simulink model "Lab_5"  (R2017b)
settings: Solver=VariableStepAuto  StartTime=0.0  StopTime=inf  MaxStep=0.1
values from neighbouring files (symbols this model uses):
  a = (r_a + r_p)/2    (= 7975.5)    [main.m]
  A_i = [A_i_1, A_i_2, A_i_3]    [main.m]
  alpha_m = deg2rad(11)    [main.m]
  C_d = 2.2    [main.m]
  DCM_0 = eye(3)    [main.m]
  dim = [w, l, h]    [main.m]
  i = 0    [main.m]
  I_1 = M/12 * (w^2 + l^2)    (= 0.0153029225)    [main.m]
  I_2 = M/12 * (w^2 + h^2)    (= 0.0314850625)    [main.m]
  I_3 = M/12 * (l^2 + h^2)    (= 0.041787985)    [main.m]
  m_m = (a_m^3*H_0)*(4*pi/mu_0)    [main.m]
  mu = 398600    [main.m]
  n = 2*pi/(60*60*24*365)    (= 1.99238499086e-07)    [main.m]
  OMG = 0    [main.m]
  omg = 0    [main.m]
  phi_0 = 0.1    [main.m]
  psi_0 = 0.1    [main.m]
  q_0 = [0 1/sqrt(3) 1/sqrt(3) 1/sqrt(3)]    [main.m]
  q_c = [0 0 0 1]'    [main.m]
  R_e = 6.378e+03    (= 6378)    [main.m]
  rho_d = 0.1    [main.m]
  rho_s = 0.5    [main.m]
  theta = 0    [main.m]
  theta_0 = 0.1    [main.m]
  w1_0 = 0    [main.m]
  w2_0 = 0    [main.m]
  w3_0 = (sqrt(mu/(7.9755e+03)^3))/10    [main.m]
  w_e = [0 0 0.00007291]    [main.m]
libraries: simulink x2, vrlib x2, dspmathops x2, sharedutil x1
settings Model: Creator=fcuzzocrea  LastModifiedBy=fcuzzocrea

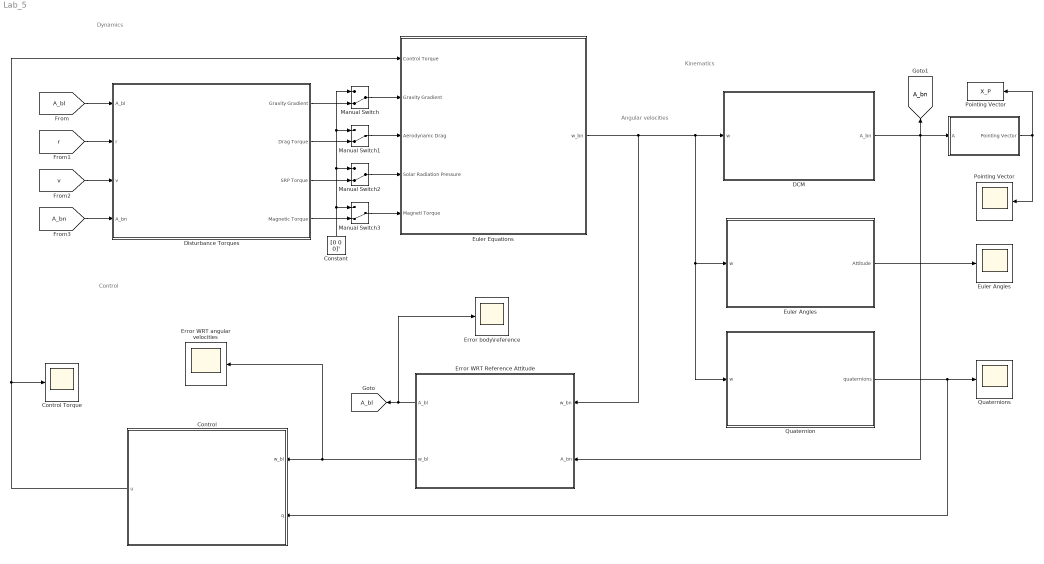
== system Lab_5 ==
  note: Control
  note: Dynamics
  note: Kinematics
  note: Angular velocities
  " " : Subsystem
  Constant : Constant  Value=[0 0 0]'
  Control : Subsystem
  "Control Torque " : Scope
  DCM : Subsystem
  Disturbance Torques : Subsystem
  "Error WRT Reference Attitude " : Subsystem
  Error WRT angular velocities : Scope
  "Error body\\reference  " : Scope
  "Euler Angles " : Subsystem
  "Euler Angles " : Scope
  "Euler Equations " : Subsystem
  Manual Switch{,1..3} (4 alike) : ManualSwitch  CurrentSetting=0
  Pointing Vector : Scope
  "Pointing Vector " : ToWorkspace  VariableName=X_P  SampleTime=-1
  Quaternion : Subsystem
  "Quaternions " : Scope
  tag scope: A_bl=global, A_bn=global
  wires:
  DCM/1(A_bn) -> [A_bn], "Error WRT Reference Attitude "/2(A_bn), " "/1(A)
  " "/1("Pointing Vector ") -> Pointing Vector/1, "Pointing Vector "/1
  "Euler Angles "/1(Attitude) -> "Euler Angles "/1
  "Euler Equations "/1(w_bn) -> "Error WRT Reference Attitude "/1(w_bn), Quaternion/1(w), "Euler Angles "/1(w), DCM/1(w)
  [A_bl] -> Disturbance Torques/1(A_bl)
  [r] -> Disturbance Torques/2(r)
  Manual Switch/1 -> "Euler Equations "/2(Gravity Gradient)
  Disturbance Torques/1("Gravity Gradient ") -> Manual Switch/2
  Constant/1 -> Manual Switch3/1, Manual Switch/1, Manual Switch1/1, Manual Switch2/1
  Quaternion/1(quaternions) -> Control/2(q), "Quaternions "/1
  [v] -> Disturbance Torques/3(v)
  [A_bn] -> Disturbance Torques/4(A_bn)
  Disturbance Torques/2(Drag Torque) -> Manual Switch1/2
  Manual Switch1/1 -> "Euler Equations "/3(Aerodynamc Drag)
  Disturbance Torques/3(SRP Torque) -> Manual Switch2/2
  Manual Switch2/1 -> "Euler Equations "/4(Solar Radiation Pressure)
  Manual Switch3/1 -> "Euler Equations "/5(Magneti Torque)
  Disturbance Torques/4(Magnetic Torque) -> Manual Switch3/2
  "Error WRT Reference Attitude "/1(A_bl) -> "Error body\\reference  "/1, [A_bl]
  "Error WRT Reference Attitude "/2(w_bl) -> Error WRT angular velocities/1, Control/1(w_bl)
  Control/1(u) -> "Control Torque "/1, "Euler Equations "/1(Control Torque)

== system Lab_5/  ==
  A : Inport
  Constant3 : Constant  Value=[1 0 0]'  VectorParams1D=off
  Math Function : Math  Operator=transpose  SaturateOnIntegerOverflow=on
  Product1 : Product  Multiplication=Matrix(*)
  "Pointing Vector " : Outport
  wires:
  Constant3/1 -> Product1/2
  Math Function/1 -> Product1/1
  A/1 -> Math Function/1
  Product1/1 -> "Pointing Vector "/1

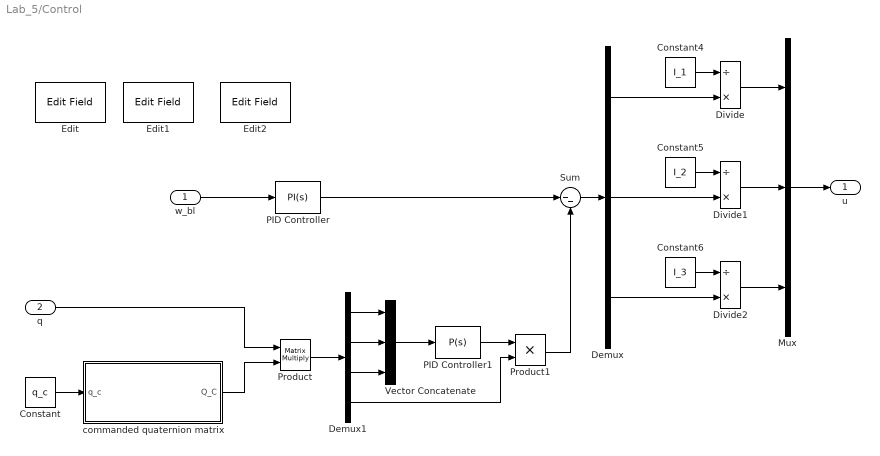
== system Lab_5/Control ==
  w_bl : Inport
  q : Inport  Port=2
  Constant : Constant  Value=q_c
  Constant4 : Constant  Value=I_1
  Constant5 : Constant  Value=I_2
  Constant6 : Constant  Value=I_3
  Demux : Demux  Outputs=3
  Demux1 : Demux
  Divide : Product  Inputs=/*
  Divide1 : Product  Inputs=/*
  Divide2 : Product  Inputs=/*
  Edit : EditField  WebBlockId=947  ModelName=Lab_5  LabelPosition=Hide  ShowInitialText=off  Alignment=Center
  Edit1 : EditField  WebBlockId=948  ModelName=Lab_5  LabelPosition=Hide  ShowInitialText=off  Alignment=Center
  Edit2 : EditField  WebBlockId=949  ModelName=Lab_5  LabelPosition=Hide  ShowInitialText=off  Alignment=Center
  Mux : Mux  Inputs=3
  PID Controller : simulink/Continuous/PID Controller  Controller=PI  TimeDomain=Continuous-time  SampleTime=-1  IntegratorMethod=Forward Euler  FilterMethod=Forward Euler  Form=Parallel  UseFilter=on  ControllerParametersSource=internal  P=1.1  I=0.3  D=0  N=100  InitialConditionSource=internal  InitialConditionForIntegrator=0  InitialConditionForFilter=0  ExternalReset=none  LimitOutput=off  UpperSaturationLimit=inf  LowerSaturationLimit=-inf  LinearizeAsGain=on  AntiWindupMode=none  Kb=1  TrackingMode=off  Kt=1  PParamMin=[]  PParamMax=[]  IParamMin=[]  IParamMax=[]  DParamMin=[]  DParamMax=[]  NParamMin=[]  NParamMax=[]  KbParamMin=[]  KbParamMax=[]  KtParamMin=[]  KtParamMax=[]  POutMin=[]  POutMax=[]  IOutMin=[]  IOutMax=[]  DOutMin=[]  DOutMax=[]  NOutMin=[]  NOutMax=[]  KbOutMin=[]  KbOutMax=[]  KtOutMin=[]  KtOutMax=[]  IntegratorOutMin=[]  IntegratorOutMax=[]  FilterOutMin=[]  FilterOutMax=[]  SumOutMin=[]  SumOutMax=[]  SumI1OutMin=[]  SumI1OutMax=[]  SumI2OutMin=[]  SumI2OutMax=[]  SumI3OutMin=[]  SumI3OutMax=[]  SumDOutMin=[]  SumDOutMax=[]  SaturationOutMin=[]  SaturationOutMax=[]  IntegratorContinuousStateAttributes=''  IntegratorStateMustResolveToSignalObject=off  IntegratorRTWStateStorageClass=Auto  FilterContinuousStateAttributes=''  FilterStateMustResolveToSignalObject=off  FilterRTWStateStorageClass=Auto  DifferentiatorICPrevScaledInput=0  DifferentiatorOutMin=[]  DifferentiatorOutMax=[]  InitialConditionSetting=State (most efficient)  FilterDiffOutCoefMin=[]  FilterDiffOutCoefMax=[]  SumDenOutMin=[]  SumDenOutMax=[]  SumNumOutMin=[]  SumNumOutMax=[]  ReciprocalOutMin=[]  ReciprocalOutMax=[]  DivideOutMin=[]  DivideOutMax=[]  TunerSelectOption=Transfer Function Based (PID Tuner App)
  PID Controller1 : simulink/Continuous/PID Controller  Controller=P  TimeDomain=Continuous-time  SampleTime=-1  IntegratorMethod=Forward Euler  FilterMethod=Forward Euler  Form=Parallel  UseFilter=on  ControllerParametersSource=internal  P=0.001  I=0.1e-3  D=0  N=100  InitialConditionSource=internal  InitialConditionForIntegrator=0  InitialConditionForFilter=0  ExternalReset=none  LimitOutput=off  UpperSaturationLimit=inf  LowerSaturationLimit=-inf  LinearizeAsGain=on  AntiWindupMode=none  Kb=1  TrackingMode=off  Kt=1  PParamMin=[]  PParamMax=[]  IParamMin=[]  IParamMax=[]  DParamMin=[]  DParamMax=[]  NParamMin=[]  NParamMax=[]  KbParamMin=[]  KbParamMax=[]  KtParamMin=[]  KtParamMax=[]  POutMin=[]  POutMax=[]  IOutMin=[]  IOutMax=[]  DOutMin=[]  DOutMax=[]  NOutMin=[]  NOutMax=[]  KbOutMin=[]  KbOutMax=[]  KtOutMin=[]  KtOutMax=[]  IntegratorOutMin=[]  IntegratorOutMax=[]  FilterOutMin=[]  FilterOutMax=[]  SumOutMin=[]  SumOutMax=[]  SumI1OutMin=[]  SumI1OutMax=[]  SumI2OutMin=[]  SumI2OutMax=[]  SumI3OutMin=[]  SumI3OutMax=[]  SumDOutMin=[]  SumDOutMax=[]  SaturationOutMin=[]  SaturationOutMax=[]  IntegratorContinuousStateAttributes=''  IntegratorStateMustResolveToSignalObject=off  IntegratorRTWStateStorageClass=Auto  FilterContinuousStateAttributes=''  FilterStateMustResolveToSignalObject=off  FilterRTWStateStorageClass=Auto  DifferentiatorICPrevScaledInput=0  DifferentiatorOutMin=[]  DifferentiatorOutMax=[]  InitialConditionSetting=State (most efficient)  FilterDiffOutCoefMin=[]  FilterDiffOutCoefMax=[]  SumDenOutMin=[]  SumDenOutMax=[]  SumNumOutMin=[]  SumNumOutMax=[]  ReciprocalOutMin=[]  ReciprocalOutMax=[]  DivideOutMin=[]  DivideOutMax=[]  TunerSelectOption=Transfer Function Based (PID Tuner App)
  Product : Product  Multiplication=Matrix(*)
  Product1 : Product
  Sum : Sum  Inputs=|--
  Vector Concatenate : Concatenate  NumInputs=3
  commanded quaternion matrix : MATLAB Function  TreatAsAtomicUnit=on
  u : Outport
  wires:
  w_bl/1 -> PID Controller/1
  Divide/1 -> Mux/1
  Constant4/1 -> Divide/1
  Constant5/1 -> Divide1/1
  Divide1/1 -> Mux/2
  Constant6/1 -> Divide2/1
  Divide2/1 -> Mux/3
  Demux/2 -> Divide1/2
  Demux/1 -> Divide/2
  Mux/1 -> u/1
  Demux/3 -> Divide2/2
  Constant/1 -> commanded quaternion matrix/1(q_c)
  q/1 -> Product/1
  commanded quaternion matrix/1(Q_C) -> Product/2
  PID Controller/1 -> Sum/1
  Sum/1 -> Demux/1
  Product/1 -> Demux1/1
  Demux1/4 -> Product1/2
  Demux1/1 -> Vector Concatenate/1
  Demux1/2 -> Vector Concatenate/2
  Demux1/3 -> Vector Concatenate/3
  Vector Concatenate/1 -> PID Controller1/1
  PID Controller1/1 -> Product1/1
  Product1/1 -> Sum/2

== system Lab_5/DCM ==
  w : Inport  Unit=rad/s  PortDimensions=3
  fromBodyToEarth : Subsystem
  A_bn : Outport
  wires:
  w/1 -> fromBodyToEarth/1("w ")
  fromBodyToEarth/1(A_bn) -> A_bn/1

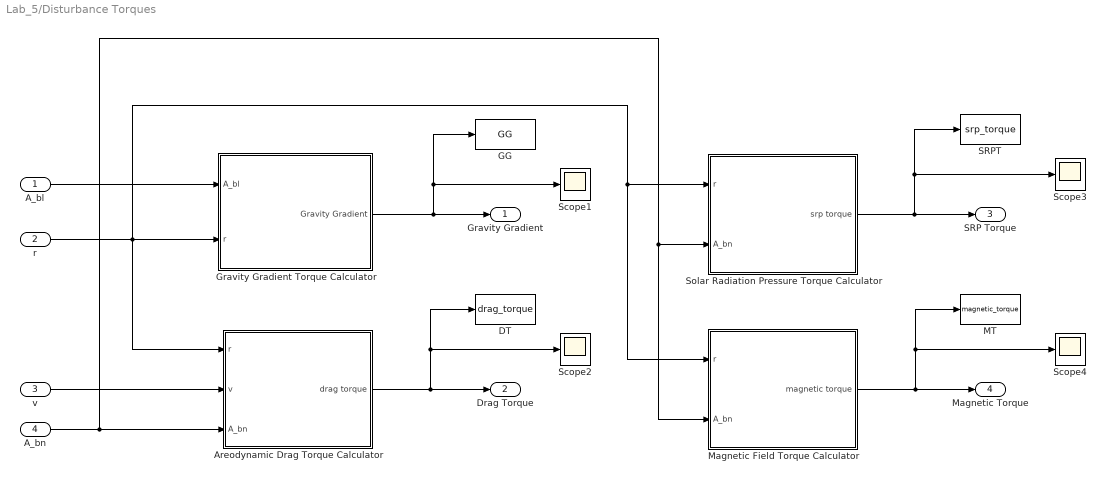
== system Lab_5/Disturbance Torques ==
  A_bl : Inport
  r : Inport  Port=2
  v : Inport  Port=3
  A_bn : Inport  Port=4
  "Areodynamic Drag Torque Calculator " : Subsystem
  DT : ToWorkspace  VariableName=drag_torque  SampleTime=-1
  GG : ToWorkspace  VariableName=GG  SampleTime=-1
  Gravity Gradient Torque Calculator : Subsystem
  MT : ToWorkspace  VariableName=magnetic_torque  SampleTime=-1
  Magnetic Field Torque Calculator : Subsystem
  SRPT : ToWorkspace  VariableName=srp_torque  SampleTime=-1
  Scope{1..4} (4 alike) : Scope
  Solar Radiation Pressure Torque Calculator : Subsystem
  "Gravity Gradient " : Outport
  Drag Torque : Outport  Port=2
  SRP Torque : Outport  Port=3
  Magnetic Torque : Outport  Port=4
  wires:
  A_bl/1 -> Gravity Gradient Torque Calculator/1(A_bl)
  Gravity Gradient Torque Calculator/1(Gravity Gradient) -> GG/1, Scope1/1, "Gravity Gradient "/1
  v/1 -> "Areodynamic Drag Torque Calculator "/2(v)
  A_bn/1 -> Magnetic Field Torque Calculator/2(A_bn), Solar Radiation Pressure Torque Calculator/2(A_bn), "Areodynamic Drag Torque Calculator "/3(A_bn)
  "Areodynamic Drag Torque Calculator "/1("drag torque ") -> DT/1, Scope2/1, Drag Torque/1
  Solar Radiation Pressure Torque Calculator/1("srp torque ") -> SRP Torque/1, Scope3/1, SRPT/1
  Magnetic Field Torque Calculator/1("magnetic torque ") -> Magnetic Torque/1, Scope4/1, MT/1
  r/1 -> "Areodynamic Drag Torque Calculator "/1(r), Gravity Gradient Torque Calculator/2(r), Magnetic Field Torque Calculator/1(r), Solar Radiation Pressure Torque Calculator/1(r)

== system Lab_5/Error WRT Reference Attitude  ==
  note: Error on angular velocities
  note: Error on reference frames
  note: OSS : Reference frame here stands for frame that we wan to track, don't make confusion
  w_bn : Inport
  A_bn : Inport  Port=2
  Angular velocity of the orbital pointing frame : Subsystem
  Relative angular velocities between the body frame and the orbital pointing frame (the error in terms of angular velocities). : Subsystem
  Rotation matrix between the body frame and the orbital pointing frame (the error on pointing) : Subsystem
  To Workspace : ToWorkspace  VariableName=w_bl  SampleTime=-1
  A_bl : Outport
  w_bl : Outport  Port=2
  wires:
  A_bn/1 -> Rotation matrix between the body frame and the orbital pointing frame (the error on pointing)/1("A_bn ")
  w_bn/1 -> Relative angular velocities between the body frame and the orbital pointing frame (the error in terms of angular velocities)./1(w_bn)
  Rotation matrix between the body frame and the orbital pointing frame (the error on pointing)/1("A_bl ") -> A_bl/1, Relative angular velocities between the body frame and the orbital pointing frame (the error in terms of angular velocities)./2("A_bl ")
  Angular velocity of the orbital pointing frame/1(w_ln) -> Relative angular velocities between the body frame and the orbital pointing frame (the error in terms of angular velocities)./3("w_ln ")
  Relative angular velocities between the body frame and the orbital pointing frame (the error in terms of angular velocities)./1(w_bl) -> To Workspace/1, w_bl/1

== system Lab_5/Euler Angles  ==
  w : Inport
  Demux : Demux  Outputs=3
  Integrator : Integrator  InitialCondition=phi_0
  Integrator1 : Integrator  InitialCondition=theta_0
  Integrator2 : Integrator  InitialCondition=psi_0
  MATLAB Function : MATLAB Function  TreatAsAtomicUnit=on
  Mux : Mux  Inputs=3
  Attitude : Outport
  wires:
  Demux/1 -> MATLAB Function/1(w1)
  Demux/2 -> MATLAB Function/2(w2)
  Demux/3 -> MATLAB Function/3(w3)
  MATLAB Function/1(phi_dot) -> Integrator/1
  MATLAB Function/2(tetha_dot) -> Integrator1/1
  MATLAB Function/3(psi_dot) -> Integrator2/1
  Integrator/1 -> Mux/1
  Integrator1/1 -> Mux/2, MATLAB Function/4(tetha)
  Mux/1 -> Attitude/1
  Integrator2/1 -> MATLAB Function/5(psi), Mux/3
  w/1 -> Demux/1

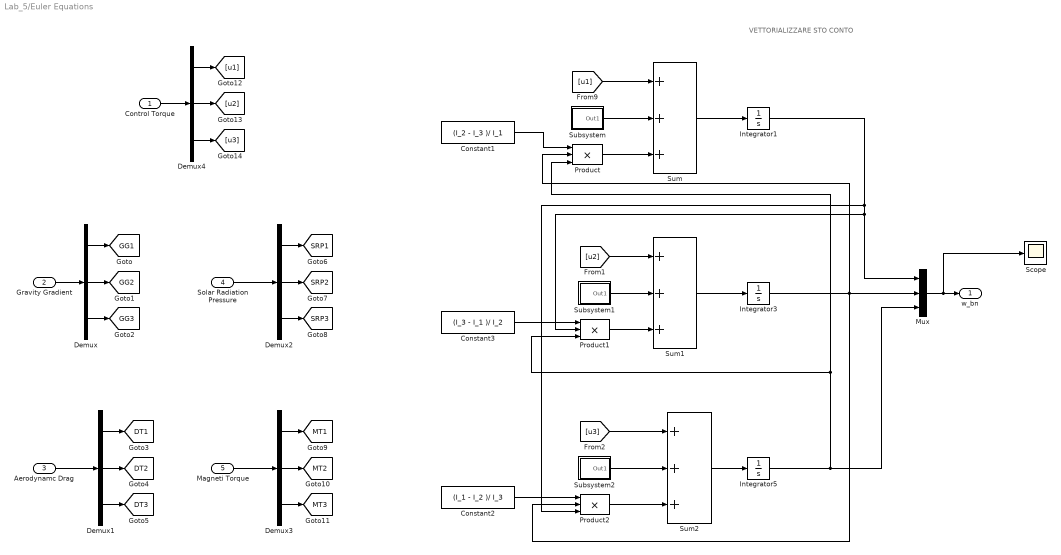
== system Lab_5/Euler Equations  ==
  note: VETTORIALIZZARE STO CONTO
  Control Torque : Inport
  Gravity Gradient : Inport  Port=2
  Aerodynamc Drag : Inport  Port=3
  Solar Radiation Pressure : Inport  Port=4
  Magneti Torque : Inport  Port=5
  Constant1 : Constant  Value=(I_2 - I_3 )/ I_1
  Constant2 : Constant  Value=(I_1 - I_2 )/ I_3
  Constant3 : Constant  Value=(I_3 - I_1 )/ I_2
  Demux{,1..4} (5 alike) : Demux  Outputs=3
  Integrator1 : Integrator  InitialCondition=w1_0
  Integrator3 : Integrator  InitialCondition=w2_0
  Integrator5 : Integrator  InitialCondition=w3_0
  Mux : Mux  Inputs=3
  Product : Product  Inputs=3
  Product1 : Product  Inputs=3
  Product2 : Product  Inputs=3
  Scope : Scope
  Subsystem : Subsystem
  Subsystem1 : Subsystem
  Subsystem2 : Subsystem
  Sum : Sum  Inputs=+++
  Sum1 : Sum  Inputs=+++
  Sum2 : Sum  Inputs=+++
  w_bn : Outport  Unit=rad/s  PortDimensions=3
  tag scope: DT1=global, DT2=global, DT3=global, GG1=global, GG2=global, GG3=global, MT1=global, MT2=global, MT3=global, SRP1=global, SRP2=global, SRP3=global
  wires:
  Integrator3/1 -> Product2/2, Mux/2, Product/2
  Integrator5/1 -> Product/3, Product1/3, Mux/3
  Constant1/1 -> Product/1
  Constant3/1 -> Product1/1
  Constant2/1 -> Product2/1
  Integrator1/1 -> Mux/1, Product1/2, Product2/3
  Mux/1 -> w_bn/1, Scope/1
  Gravity Gradient/1 -> Demux/1
  Demux/1 -> [GG1]
  Demux/2 -> [GG2]
  Demux/3 -> [GG3]
  Demux1/3 -> [DT3]
  Aerodynamc Drag/1 -> Demux1/1
  Demux1/2 -> [DT2]
  Demux1/1 -> [DT1]
  Demux2/3 -> [SRP3]
  Solar Radiation Pressure/1 -> Demux2/1
  Demux2/1 -> [SRP1]
  Demux2/2 -> [SRP2]
  Demux3/2 -> [MT2]
  Demux3/3 -> [MT3]
  Demux3/1 -> [MT1]
  Magneti Torque/1 -> Demux3/1
  Demux4/1 -> [u1]
  Demux4/3 -> [u3]
  Control Torque/1 -> Demux4/1
  Demux4/2 -> [u2]
  Subsystem/1(Out1) -> Sum/2
  Product/1 -> Sum/3
  Sum/1 -> Integrator1/1
  Sum1/1 -> Integrator3/1
  Product1/1 -> Sum1/3
  Subsystem1/1(Out1) -> Sum1/2
  Sum2/1 -> Integrator5/1
  Product2/1 -> Sum2/3
  Subsystem2/1(Out1) -> Sum2/2
  [u1] -> Sum/1
  [u3] -> Sum2/1
  [u2] -> Sum1/1

== system Lab_5/Quaternion ==
  w : Inport
  Integrator2 : Integrator  InitialCondition=q_0
  Quaternion kinematics : MATLAB Function  TreatAsAtomicUnit=on
  quaternions : Outport
  wires:
  Integrator2/1 -> quaternions/1, Quaternion kinematics/1(q)  "q"
  Quaternion kinematics/1(dq) -> Integrator2/1  "dq"
  w/1 -> Quaternion kinematics/2(omega)  "ω_b"

== system Lab_5/DCM/fromBodyToEarth ==
  "w " : Inport
  "Assembly [w^] " : Subsystem
  Demux : Demux  Outputs=3
  Integrator : Integrator  InitialCondition=DCM_0
  MATLAB Function1 : MATLAB Function  TreatAsAtomicUnit=on
  Product : Product  Multiplication=Matrix(*)
  A_bn : Outport
  wires:
  Product/1 -> Integrator/1
  Integrator/1 -> A_bn/1, MATLAB Function1/1(u)
  "w "/1 -> Demux/1
  Demux/1 -> "Assembly [w^] "/1(w1)
  Demux/2 -> "Assembly [w^] "/2(w2)
  Demux/3 -> "Assembly [w^] "/3(w3)
  "Assembly [w^] "/1(-[w]^) -> Product/1
  MATLAB Function1/1(y) -> Product/2

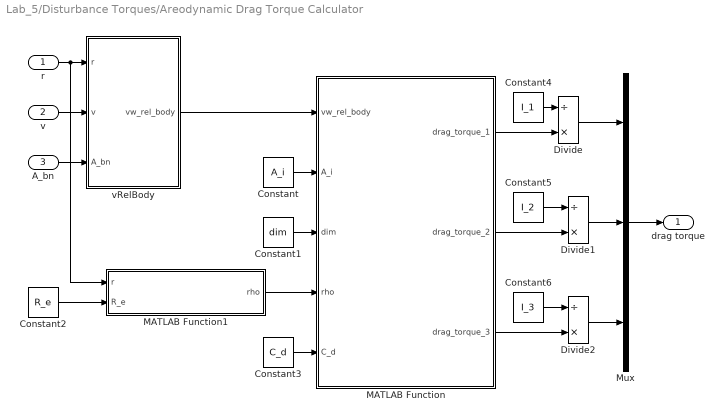
== system Lab_5/Disturbance Torques/Areodynamic Drag Torque Calculator  ==
  r : Inport
  v : Inport  Port=2
  A_bn : Inport  Port=3
  Constant : Constant  Value=A_i
  Constant1 : Constant  Value=dim
  Constant2 : Constant  Value=R_e
  Constant3 : Constant  Value=C_d
  Constant4 : Constant  Value=I_1
  Constant5 : Constant  Value=I_2
  Constant6 : Constant  Value=I_3
  Divide : Product  Inputs=/*
  Divide1 : Product  Inputs=/*
  Divide2 : Product  Inputs=/*
  MATLAB Function : MATLAB Function  TreatAsAtomicUnit=on
  MATLAB Function1 : MATLAB Function  TreatAsAtomicUnit=on
  Mux : Mux  Inputs=3
  vRelBody : Subsystem
  "drag torque " : Outport
  wires:
  r/1 -> MATLAB Function1/1(r), vRelBody/1(r)
  v/1 -> vRelBody/2(v)
  A_bn/1 -> vRelBody/3(A_bn)
  vRelBody/1(vw_rel_body) -> MATLAB Function/1(vw_rel_body)
  Constant/1 -> MATLAB Function/2(A_i)
  Constant1/1 -> MATLAB Function/3(dim)
  Constant3/1 -> MATLAB Function/5(C_d)
  Mux/1 -> "drag torque "/1
  MATLAB Function/1(drag_torque_1) -> Divide/2
  Divide/1 -> Mux/1
  Constant4/1 -> Divide/1
  Constant5/1 -> Divide1/1
  MATLAB Function/2(drag_torque_2) -> Divide1/2
  Divide1/1 -> Mux/2
  Constant6/1 -> Divide2/1
  MATLAB Function/3(drag_torque_3) -> Divide2/2
  Divide2/1 -> Mux/3
  Constant2/1 -> MATLAB Function1/2(R_e)
  MATLAB Function1/1(rho) -> MATLAB Function/4(rho)

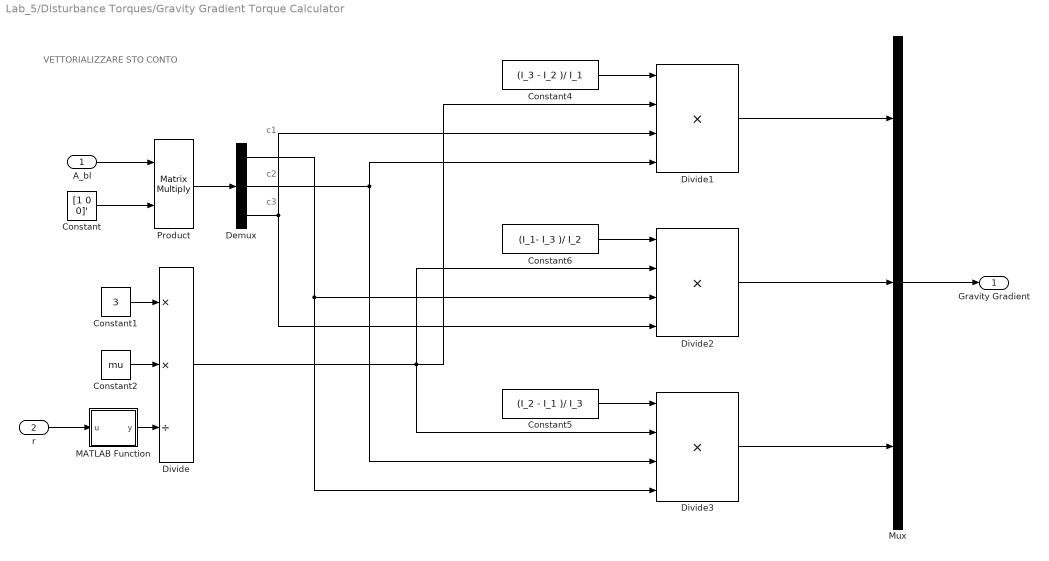
== system Lab_5/Disturbance Torques/Gravity Gradient Torque Calculator ==
  note: VETTORIALIZZARE STO CONTO
  note: c2
  note: c3
  note: c1
  A_bl : Inport
  r : Inport  Port=2
  Constant : Constant  Value=[1 0 0]'
  Constant1 : Constant  Value=3
  Constant2 : Constant  Value=mu
  Constant4 : Constant  Value=(I_3 - I_2 )/ I_1
  Constant5 : Constant  Value=(I_2 - I_1 )/ I_3
  Constant6 : Constant  Value=(I_1- I_3 )/ I_2
  Demux : Demux  Outputs=3
  Divide : Product  Inputs=**/
  Divide1 : Product  Inputs=****
  Divide2 : Product  Inputs=****
  Divide3 : Product  Inputs=****
  MATLAB Function : MATLAB Function  TreatAsAtomicUnit=on
  Mux : Mux  Inputs=3
  Product : Product  Multiplication=Matrix(*)
  Gravity Gradient : Outport
  wires:
  Demux/3 -> Divide2/4, Divide1/3
  Constant1/1 -> Divide/1
  r/1 -> MATLAB Function/1(u)
  Constant5/1 -> Divide3/1
  Divide/1 -> Divide3/2, Divide1/2, Divide2/2
  Demux/1 -> Divide3/4, Divide2/3
  Demux/2 -> Divide3/3, Divide1/4
  Product/1 -> Demux/1
  Constant6/1 -> Divide2/1
  A_bl/1 -> Product/1
  Constant4/1 -> Divide1/1
  MATLAB Function/1(y) -> Divide/3
  Constant/1 -> Product/2
  Constant2/1 -> Divide/2
  Divide1/1 -> Mux/1
  Divide2/1 -> Mux/2
  Divide3/1 -> Mux/3
  Mux/1 -> Gravity Gradient/1

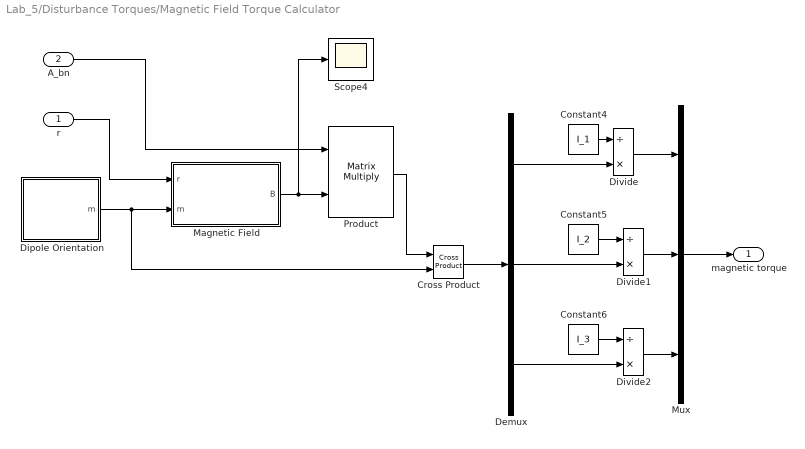
== system Lab_5/Disturbance Torques/Magnetic Field Torque Calculator ==
  r : Inport
  A_bn : Inport  Port=2
  Constant4 : Constant  Value=I_1
  Constant5 : Constant  Value=I_2
  Constant6 : Constant  Value=I_3
  Cross Product : vrlib/Utilities/Cross Product
      settings: SourceProductBaseCode=VR
  Demux : Demux  Outputs=3
  Dipole Orientation : Subsystem
  Divide : Product  Inputs=/*
  Divide1 : Product  Inputs=/*
  Divide2 : Product  Inputs=/*
  Magnetic Field : Subsystem
  Mux : Mux  Inputs=3
  Product : Product  Multiplication=Matrix(*)
  Scope4 : Scope
  "magnetic torque " : Outport
  wires:
  r/1 -> Magnetic Field/1(r)
  Demux/3 -> Divide2/2
  Mux/1 -> "magnetic torque "/1
  A_bn/1 -> Product/1
  Constant4/1 -> Divide/1
  Demux/2 -> Divide1/2
  Constant5/1 -> Divide1/1
  Demux/1 -> Divide/2
  Divide/1 -> Mux/1
  Product/1 -> Cross Product/1
  Divide1/1 -> Mux/2
  Cross Product/1 -> Demux/1
  Divide2/1 -> Mux/3
  Constant6/1 -> Divide2/1
  Magnetic Field/1("B ") -> Scope4/1, Product/2
  Dipole Orientation/1(m) -> Cross Product/2, Magnetic Field/2(m)

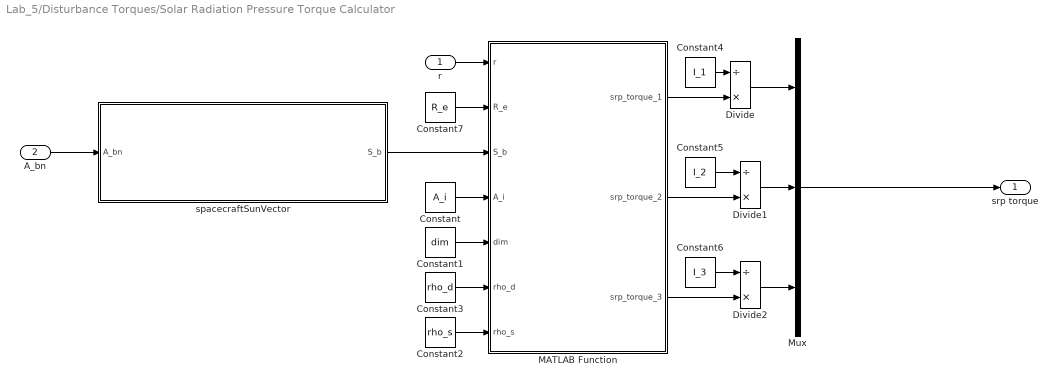
== system Lab_5/Disturbance Torques/Solar Radiation Pressure Torque Calculator ==
  r : Inport
  A_bn : Inport  Port=2
  Constant : Constant  Value=A_i
  Constant1 : Constant  Value=dim
  Constant2 : Constant  Value=rho_s
  Constant3 : Constant  Value=rho_d
  Constant4 : Constant  Value=I_1
  Constant5 : Constant  Value=I_2
  Constant6 : Constant  Value=I_3
  Constant7 : Constant  Value=R_e
  Divide : Product  Inputs=/*
  Divide1 : Product  Inputs=/*
  Divide2 : Product  Inputs=/*
  MATLAB Function : MATLAB Function  TreatAsAtomicUnit=on
  Mux : Mux  Inputs=3
  spacecraftSunVector : Subsystem
  "srp torque " : Outport
  wires:
  A_bn/1 -> spacecraftSunVector/1(A_bn)
  spacecraftSunVector/1("S_b ") -> MATLAB Function/3(S_b)
  Constant/1 -> MATLAB Function/4(A_i)
  Constant1/1 -> MATLAB Function/5(dim)
  Constant3/1 -> MATLAB Function/6(rho_d)
  Constant2/1 -> MATLAB Function/7(rho_s)
  MATLAB Function/3(srp_torque_3) -> Divide2/2
  Divide/1 -> Mux/1
  MATLAB Function/2(srp_torque_2) -> Divide1/2
  Constant5/1 -> Divide1/1
  Constant6/1 -> Divide2/1
  MATLAB Function/1(srp_torque_1) -> Divide/2
  Divide1/1 -> Mux/2
  Constant4/1 -> Divide/1
  Mux/1 -> "srp torque "/1
  Divide2/1 -> Mux/3
  r/1 -> MATLAB Function/1(r)
  Constant7/1 -> MATLAB Function/2(R_e)

== system Lab_5/Error WRT Reference Attitude /Angular velocity of the orbital pointing frame ==
  Derivative : Derivative
  MATLAB Function : MATLAB Function  TreatAsAtomicUnit=on
  Math Function : Math  Operator=transpose  SaturateOnIntegerOverflow=on
  Product : Product  Multiplication=Matrix(*)
  w_ln : Outport
  wires:
  [A_ln] -> Math Function/1, Derivative/1
  Math Function/1 -> Product/2
  Derivative/1 -> Product/1
  Product/1 -> MATLAB Function/1(w_ln_cross)
  MATLAB Function/1(w_ln) -> w_ln/1

== system Lab_5/Error WRT Reference Attitude /Relative angular velocities between the body frame and the orbital pointing frame (the error in terms of angular velocities). ==
  w_bn : Inport
  "A_bl " : Inport  Port=2
  "w_ln " : Inport  Port=3
  Product : Product  Multiplication=Matrix(*)
  Subtract : Sum  Inputs=+-
  w_bl : Outport
  wires:
  Product/1 -> Subtract/2
  Subtract/1 -> w_bl/1
  w_bn/1 -> Subtract/1
  "A_bl "/1 -> Product/1
  "w_ln "/1 -> Product/2

== system Lab_5/Error WRT Reference Attitude /Rotation matrix between the body frame and the orbital pointing frame (the error on pointing) ==
  note: NB : La DCM è A_bn, per cui moltiplicando A_ln * A_bn becco A_bl !!!!
  note: Reference Attitude
  "A_bn " : Inport
  Math Function1 : Math  Operator=transpose  SaturateOnIntegerOverflow=on
  Product : Product  Multiplication=Matrix(*)
  Rotation matrix between the pointing orbital frame and the inertial frame : Subsystem
  "A_bl " : Outport
  wires:
  "A_bn "/1 -> Product/1
  Rotation matrix between the pointing orbital frame and the inertial frame/1("A_L\\N ") -> Math Function1/1
  Product/1 -> "A_bl "/1
  Math Function1/1 -> Product/2

== system Lab_5/Euler Equations /Subsystem ==
  Sum : Sum  Inputs=++++
  Out1 : Outport
  wires:
  Sum/1 -> Out1/1
  [GG1] -> Sum/4
  [DT1] -> Sum/3
  [SRP1] -> Sum/2
  [MT1] -> Sum/1

== system Lab_5/Euler Equations /Subsystem1 ==
  Sum2 : Sum  Inputs=++++
  Out1 : Outport
  wires:
  Sum2/1 -> Out1/1
  [GG2] -> Sum2/4
  [DT2] -> Sum2/3
  [SRP2] -> Sum2/2
  [MT2] -> Sum2/1

== system Lab_5/Euler Equations /Subsystem2 ==
  Sum3 : Sum  Inputs=++++
  Out1 : Outport
  wires:
  Sum3/1 -> Out1/1
  [GG3] -> Sum3/4
  [DT3] -> Sum3/3
  [SRP3] -> Sum3/2
  [MT3] -> Sum3/1

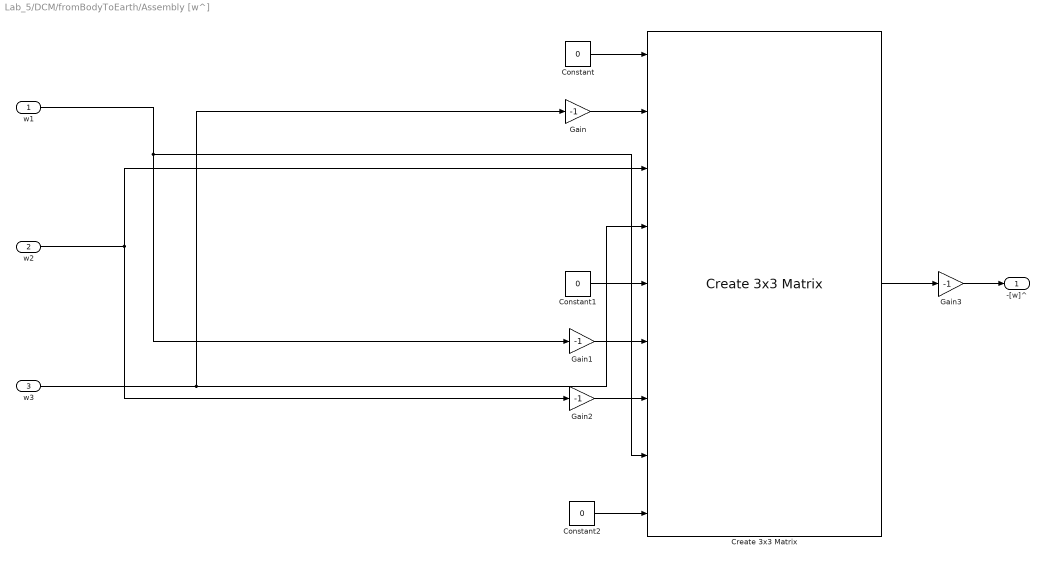
== system Lab_5/DCM/fromBodyToEarth/Assembly [w^]  ==
  w1 : Inport
  w2 : Inport  Port=2
  w3 : Inport  Port=3
  Constant : Constant  Value=0
  Constant1 : Constant  Value=0
  Constant2 : Constant  Value=0
  Create 3x3 Matrix : sharedutil/Create 3x3 Matrix
  Gain{,1..3} (4 alike) : Gain  Gain=-1
  -[w]^ : Outport
  wires:
  Gain2/1 -> Create 3x3 Matrix/7
  Gain1/1 -> Create 3x3 Matrix/6
  w1/1 -> Create 3x3 Matrix/8, Gain1/1
  w3/1 -> Create 3x3 Matrix/4, Gain/1
  Constant1/1 -> Create 3x3 Matrix/5
  Constant2/1 -> Create 3x3 Matrix/9
  Constant/1 -> Create 3x3 Matrix/1
  w2/1 -> Gain2/1, Create 3x3 Matrix/3
  Gain/1 -> Create 3x3 Matrix/2
  Create 3x3 Matrix/1 -> Gain3/1
  Gain3/1 -> -[w]^/1

== system Lab_5/Disturbance Torques/Areodynamic Drag Torque Calculator /vRelBody ==
  r : Inport
  v : Inport  Port=2
  A_bn : Inport  Port=3
  Add : Sum  Inputs=+-
  Constant : Constant  Value=w_e
  Cross Product : vrlib/Utilities/Cross Product
      settings: SourceProductBaseCode=VR
  Product : Product  Multiplication=Matrix(*)
  vw_rel_body : Outport
  wires:
  Add/1 -> Product/2
  Constant/1 -> Cross Product/1
  r/1 -> Cross Product/2
  Product/1 -> vw_rel_body/1
  v/1 -> Add/1
  A_bn/1 -> Product/1
  Cross Product/1 -> Add/2

== system Lab_5/Disturbance Torques/Magnetic Field Torque Calculator/Dipole Orientation ==
  Constant : Constant  Value=sin(alpha_m)
  Constant1 : Constant  Value=cos(alpha_m)
  Cosine Wave : Sin  Frequency=w_e(3)  Phase=pi/2  SampleTime=0
  Product : Product
  Product1 : Product
  Sine Wave : Sin  Frequency=w_e(3)  SampleTime=0
  Vector Concatenate : Concatenate  NumInputs=3
  m : Outport
  wires:
  Product/1 -> Vector Concatenate/2
  Vector Concatenate/1 -> m/1
  Cosine Wave/1 -> Product1/2
  Sine Wave/1 -> Product/2
  Constant1/1 -> Vector Concatenate/3
  Product1/1 -> Vector Concatenate/1
  Constant/1 -> Product/1, Product1/1

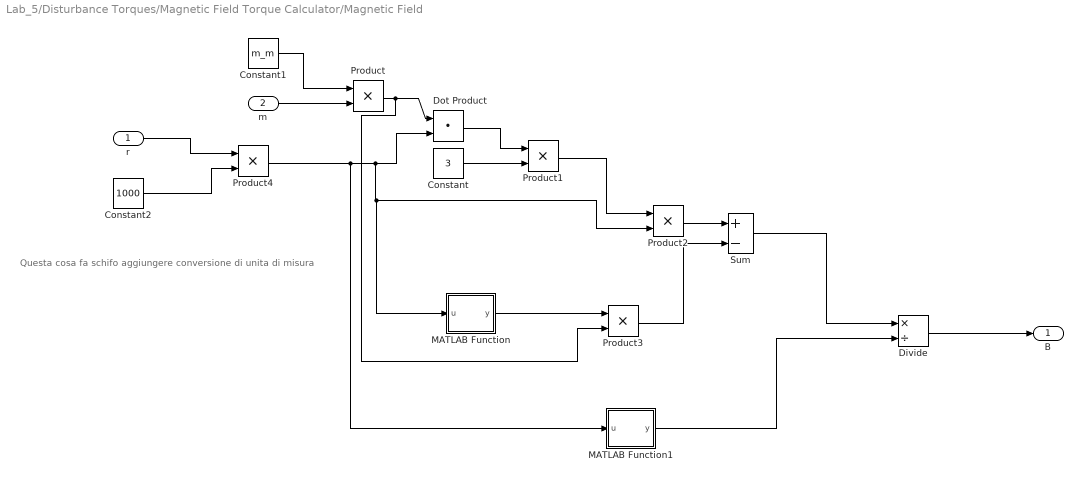
== system Lab_5/Disturbance Torques/Magnetic Field Torque Calculator/Magnetic Field ==
  note: Questa cosa fa schifo aggiungere conversione di unita di misura
  r : Inport  Unit=km
  m : Inport  Port=2
  Constant : Constant  Value=3
  Constant1 : Constant  Value=m_m
  Constant2 : Constant  Value=1000
  Divide : Product  Inputs=*/
  Dot Product : DotProduct  InputSameDT=on  OutDataTypeStr=Inherit: Inherit via internal rule
  MATLAB Function : MATLAB Function  TreatAsAtomicUnit=on
  MATLAB Function1 : MATLAB Function  TreatAsAtomicUnit=on
  Product{,1..4} (5 alike) : Product
  Sum : Sum  Inputs=+-
  "B " : Outport
  wires:
  MATLAB Function1/1(y) -> Divide/2
  Sum/1 -> Divide/1
  Product3/1 -> Sum/2
  MATLAB Function/1(y) -> Product3/1
  Product2/1 -> Sum/1
  Product1/1 -> Product2/1
  Constant/1 -> Product1/2
  Dot Product/1 -> Product1/1
  Product4/1 -> Dot Product/2, Product2/2, MATLAB Function/1(u), MATLAB Function1/1(u)
  Product/1 -> Dot Product/1, Product3/2
  Divide/1 -> "B "/1
  m/1 -> Product/2
  Constant1/1 -> Product/1
  r/1 -> Product4/1
  Constant2/1 -> Product4/2

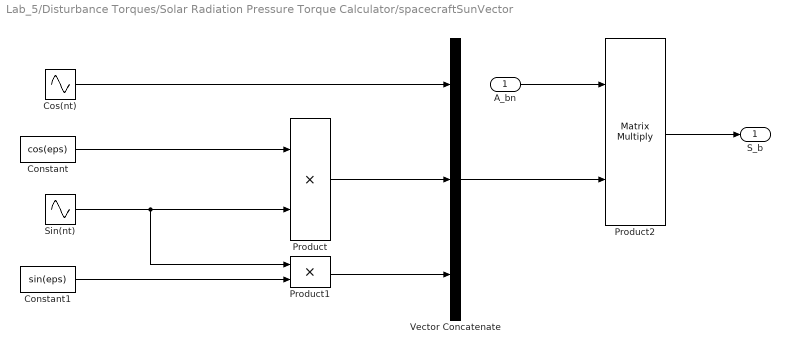
== system Lab_5/Disturbance Torques/Solar Radiation Pressure Torque Calculator/spacecraftSunVector ==
  A_bn : Inport
  Constant : Constant  Value=cos(eps)
  Constant1 : Constant  Value=sin(eps)
  Cos(nt) : Sin  Frequency=n  Phase=pi/2  SampleTime=0
  Product : Product
  Product1 : Product
  Product2 : Product  Multiplication=Matrix(*)
  Sin(nt) : Sin  Frequency=n  SampleTime=0
  Vector Concatenate : Concatenate  NumInputs=3
  "S_b " : Outport
  wires:
  Product2/1 -> "S_b "/1
  Constant/1 -> Product/1
  Constant1/1 -> Product1/2
  Sin(nt)/1 -> Product1/1, Product/2
  Product1/1 -> Vector Concatenate/3
  Vector Concatenate/1 -> Product2/2
  A_bn/1 -> Product2/1
  Product/1 -> Vector Concatenate/2
  Cos(nt)/1 -> Vector Concatenate/1

== system Lab_5/Error WRT Reference Attitude /Rotation matrix between the body frame and the orbital pointing frame (the error on pointing)/Rotation matrix between the pointing orbital frame and the inertial frame ==
  Full Orbital Dynamics : Subsystem
  Initial Conditions (KEP) : Constant  Value=[a, e, i, OMG, omg, theta]
  Planetary Constant : Constant  Value=mu
  "A_L\\N " : Outport
  tag scope: A_ln=global
  wires:
  Planetary Constant/1 -> Full Orbital Dynamics/1(mu)
  Initial Conditions (KEP)/1 -> Full Orbital Dynamics/2(Initial Condition (kep))
  Full Orbital Dynamics/1(A_L\N) -> [A_ln], "A_L\\N "/1

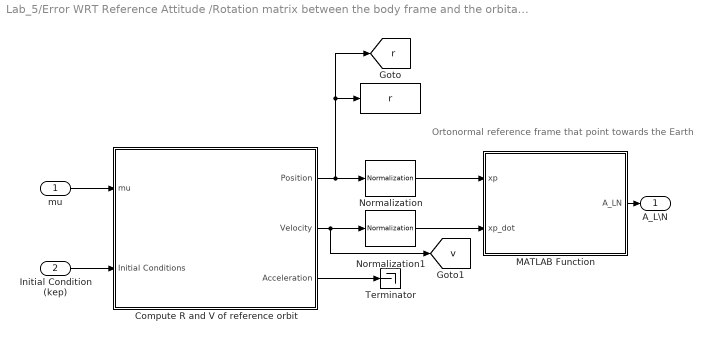
== system Lab_5/Error WRT Reference Attitude /Rotation matrix between the body frame and the orbital pointing frame (the error on pointing)/Rotation matrix between the pointing orbital frame and the inertial frame/Full Orbital Dynamics ==
  note: Ortonormal reference frame that point towards the Earth
  mu : Inport
  Initial Condition (kep) : Inport  Port=2
  " " : ToWorkspace  VariableName=r  SampleTime=-1
  Compute R and V of reference orbit : Subsystem
  MATLAB Function : MATLAB Function  TreatAsAtomicUnit=on
  Normalization : dspmathops/Normalization  NormType=2-norm  Bias=1e-10  NormOver=Each row  Dimension=1  outputDataTypeStr=Inherit: Same as product output  outputLastDataTypeStr=Inherit: Same as product output  outputMin=[]  outputMax=[]  accumDataTypeStr=Inherit: Same as product output  accumLastDataTypeStr=Inherit: Same as product output  roundingMode=Floor  overflowMode=off
      settings: SourceProductName=DSP System Toolbox
  Normalization1 : dspmathops/Normalization  NormType=2-norm  Bias=1e-10  NormOver=Each row  Dimension=1  outputDataTypeStr=Inherit: Same as product output  outputLastDataTypeStr=Inherit: Same as product output  outputMin=[]  outputMax=[]  accumDataTypeStr=Inherit: Same as product output  accumLastDataTypeStr=Inherit: Same as product output  roundingMode=Floor  overflowMode=off
      settings: SourceProductName=DSP System Toolbox
  Terminator : Terminator
  A_L\N : Outport
  tag scope: r=global, v=global
  wires:
  mu/1 -> Compute R and V of reference orbit/1(mu)
  Initial Condition (kep)/1 -> Compute R and V of reference orbit/2(Initial Conditions)
  Compute R and V of reference orbit/1(Position) -> [r], " "/1, Normalization/1
  Compute R and V of reference orbit/2(Velocity) -> [v], Normalization1/1
  Compute R and V of reference orbit/3(Acceleration) -> Terminator/1
  Normalization/1 -> MATLAB Function/1(xp)
  MATLAB Function/1(A_LN) -> A_L\N/1
  Normalization1/1 -> MATLAB Function/2(xp_dot)

== system Lab_5/Error WRT Reference Attitude /Rotation matrix between the body frame and the orbital pointing frame (the error on pointing)/Rotation matrix between the pointing orbital frame and the inertial frame/Full Orbital Dynamics/Compute R and V of reference orbit ==
  mu : Inport
  Initial Conditions : Inport  Port=2
  Initial Position : Subsystem
  Initial Velocity : Subsystem
  Integrator : Integrator  InitialConditionSource=external  InitialCondition=[r,v]=kep2car(kep,mu);  ContinuousStateAttributes='velocity'
  Integrator2 : Integrator  InitialConditionSource=external  InitialCondition=[r,v]=kep2car(kep,mu);  ContinuousStateAttributes='position'
  Orbital Dynamics : MATLAB Function  TreatAsAtomicUnit=on
  Position : Outport
  Velocity : Outport  Port=2
  Acceleration : Outport  Port=3
  wires:
  Initial Conditions/1 -> Initial Position/2(Initial Conditions), Initial Velocity/2(Initial Conditions)
  Initial Position/1(r_0) -> Integrator2/2
  Initial Velocity/1(v_0) -> Integrator/2
  Orbital Dynamics/1(a) -> Acceleration/1, Integrator/1
  Integrator/1 -> Velocity/1, Integrator2/1
  mu/1 -> Initial Position/1(mu), Initial Velocity/1(mu), Orbital Dynamics/2(mu)
  Integrator2/1 -> Orbital Dynamics/1(r), Position/1

== system Lab_5/Error WRT Reference Attitude /Rotation matrix between the body frame and the orbital pointing frame (the error on pointing)/Rotation matrix between the pointing orbital frame and the inertial frame/Full Orbital Dynamics/Compute R and V of reference orbit/Initial Position ==
  mu : Inport
  Initial Conditions : Inport  Port=2
  MATLAB Function2 : MATLAB Function  TreatAsAtomicUnit=on
  r_0 : Outport
  wires:
  MATLAB Function2/1(r_0) -> r_0/1
  mu/1 -> MATLAB Function2/2(mu)
  Initial Conditions/1 -> MATLAB Function2/1(kep)

== system Lab_5/Error WRT Reference Attitude /Rotation matrix between the body frame and the orbital pointing frame (the error on pointing)/Rotation matrix between the pointing orbital frame and the inertial frame/Full Orbital Dynamics/Compute R and V of reference orbit/Initial Velocity ==
  mu : Inport
  Initial Conditions : Inport  Port=2
  MATLAB Function1 : MATLAB Function  TreatAsAtomicUnit=on
  v_0 : Outport
  wires:
  MATLAB Function1/1(v_0) -> v_0/1
  mu/1 -> MATLAB Function1/2(mu)
  Initial Conditions/1 -> MATLAB Function1/1(kep)

== matlab function Lab_5/Euler Angles /MATLAB Function ==
  data: phi_dot output; tetha_dot output; psi_dot output; w1 input; w2 input; w3 input; tetha input; psi input
function [phi_dot,tetha_dot, psi_dot] = euler_eqtns(w1,w2,w3, tetha, psi)

% Euler rotations (sequence 123)
phi_dot = 1/cos(tetha)*((w1*cos(psi)-w2*sin(psi)));
tetha_dot = (w2*cos(psi))+(w1*sin(psi));
psi_dot = w3 - ((w1*cos(psi) - w2*sin(psi))*(sin(tetha)/cos(tetha)));

end

== matlab function Lab_5/Error WRT Reference Attitude /Rotation matrix between the body frame and the orbital pointing frame (the error on pointing)/Rotation matrix between the pointing orbital frame and the inertial frame/Full Orbital Dynamics/Compute R and V of reference orbit/Orbital Dynamics ==
  data: r input; a output; mu input
function a  = orbit_equation(r,mu)

rn = norm(r);

a = -(mu/norm(r)^3)*r;

end

== matlab function Lab_5/DCM/fromBodyToEarth/MATLAB Function1 ==
  data: u input; y output
function y = ortonormalize(u)

y = u.*3/2 - u*u'*(u./2);

y = u;

end

== matlab function Lab_5/Error WRT Reference Attitude /Rotation matrix between the body frame and the orbital pointing frame (the error on pointing)/Rotation matrix between the pointing orbital frame and the inertial frame/Full Orbital Dynamics/Compute R and V of reference orbit/Initial Velocity/MATLAB Function1 ==
  data: v_0 output; kep input; mu input
function v_0  = kep2car(kep,mu)

% Using kep2car function to find velocity at initial condition
[~,v_0]=kep2car(kep,mu);

end

== matlab function Lab_5/Error WRT Reference Attitude /Rotation matrix between the body frame and the orbital pointing frame (the error on pointing)/Rotation matrix between the pointing orbital frame and the inertial frame/Full Orbital Dynamics/Compute R and V of reference orbit/Initial Position/MATLAB Function2 ==
  data: r_0 output; kep input; mu input
function r_0  = kep2car(kep,mu)

% Using kep2car function to find position and velocity at initial condition
[r_0,~]=kep2car(kep,mu);

end

== matlab function Lab_5/Error WRT Reference Attitude /Rotation matrix between the body frame and the orbital pointing frame (the error on pointing)/Rotation matrix between the pointing orbital frame and the inertial frame/Full Orbital Dynamics/MATLAB Function ==
  data: xp input; A_LN output; xp_dot input
function A_LN = assembly_ALN(xp,xp_dot)

xp = xp';
xp_dot = xp_dot';

r_1 = xp;                                           % Points toward the Earth
r_2 = (cross(xp_dot,xp))/(norm(cross(xp_dot,xp)));  % Points toward angular momentum vector
r_3 = cross(r_1,r_2);                               % To be ortoghonal

A_LN = [r_1; r_3; r_2];                             % BE CONSISTENT WITH THE ACTUAL REFERENCE SYSTEM USED TO COMPUTE R AND V
                                                    % ACTUALLY FOR ME :
                                                    %    
                                                    %      x = direction of the vector pointing to earth    
                                                    %
                                                    %      z = direction of the out of plane vector     
                                                    %      
                                                    %      y = third vector
                                                    %

end

== matlab function Lab_5/Error WRT Reference Attitude /Angular velocity of the orbital pointing frame/MATLAB Function ==
  data: w_ln_cross input; w_ln output
function w_ln = w_component_extractor(w_ln_cross)

w_1 = w_ln_cross(3,2);
w_2 = w_ln_cross(1,3);
w_3 = w_ln_cross(2,1);

w_ln = [w_1, w_2, w_3]';
end

== matlab function Lab_5/Disturbance Torques/Gravity Gradient Torque Calculator/MATLAB Function ==
  data: u input; y output
function y = norm3(u)

y = (norm(u))^3;

end

== matlab function Lab_5/Disturbance Torques/Areodynamic Drag Torque Calculator /MATLAB Function ==
  data: vw_rel_body input; drag_torque_1 output; A_i input; dim input; rho input; C_d input; drag_torque_2 output; drag_torque_3 output
function [drag_torque_1,drag_torque_2,drag_torque_3]  = aerodrag(vw_rel_body,A_i,dim,rho, C_d)

% Velocity is in km/s, we need it in m/s
vw_rel_body = vw_rel_body .* 1e3;

% Define normal vectors
n_1 = [1 0 0];
n_2 = [0 1 0];
n_3 = [0 0 1];
n_4 = [-1 0 0];
n_5 = [0 -1 0];
n_6 = [0 0 -1];

% Dimensions 
w = dim(1);
l = dim(2);
h = dim(3);

% Sections 
A_i_1 = A_i(1);
A_i_2 = A_i(2);
A_i_3 = A_i(3);
A_i_4 = A_i(1);
A_i_5 = A_i(2);
A_i_6 = A_i(3);

% Distance between the center of pressure and the center of mass 0.1*rcg
r_1 = [h/2 0.1 0.1];
r_2 = [0.2 l/2 0.2];
r_3 = [0.4 0.4 w/2];
r_4 = [-h/2 0.1 0.1];
r_5 = [0.2 -l/2 0.2];
r_6 = [0.4 0.4 -w/2];

% Compute Aerodynamic Torque : reference Fundamentals of Spacecraft
% Dynamics and Control pag. 108
% Compute the dynamic pressure
dynamic_pressure = -0.5*rho*norm(vw_rel_body)*vw_rel_body;

% Compute torque due to the aerodynamic force only on face wetted by air
% If dot(n_1,vw_rel_body/norm(vw_rel_body)) >=0 then the face is wetted
% othewise no. 
if dot(n_1,vw_rel_body/norm(vw_rel_body)) >= 0 
    F_aero_1 = dynamic_pressure * C_d * A_i_1 * dot(n_1,vw_rel_body)/norm(vw_rel_body);
    T_aero_1 = cross(r_1,F_aero_1);
else
    T_aero_1 = [0 0 0];
end

if dot(n_2,vw_rel_body/norm(vw_rel_body)) >= 0 
    F_aero_2 = dynamic_pressure * C_d * A_i_2 * dot(n_2,vw_rel_body)/norm(vw_rel_body);
    T_aero_2 = cross(r_2,F_aero_2);
else
    T_aero_2 = [0 0 0];
end

if dot(n_3,vw_rel_body/norm(vw_rel_body)) >= 0  
    F_aero_3 = dynamic_pressure * C_d * A_i_3 * dot(n_3,vw_rel_body)/norm(vw_rel_body);
    T_aero_3 = cross(r_3,F_aero_3);
else
    T_aero_3 = [0 0 0];
end

if dot(n_4,vw_rel_body/norm(vw_rel_body)) >= 0 
    F_aero_4 = dynamic_pressure * C_d * A_i_4 * dot(n_4,vw_rel_body)/norm(vw_rel_body);
    T_aero_4 = cross(r_4,F_aero_4);
else
    T_aero_4 = [0 0 0];
end

if dot(n_5,vw_rel_body/norm(vw_rel_body)) >= 0 
    F_aero_5 = dynamic_pressure * C_d * A_i_5 * dot(n_5,vw_rel_body)/norm(vw_rel_body);
    T_aero_5 = cross(r_5,F_aero_5);
else
    T_aero_5 = [0 0 0];
end

if dot(n_6,vw_rel_body/norm(vw_rel_body)) >= 0  
    F_aero_6 = dynamic_pressure * C_d * A_i_6 * dot(n_6,vw_rel_body)/norm(vw_rel_body);
    T_aero_6 = cross(r_6,F_aero_6);
else
    T_aero_6 = [0 0 0];
end

% Sum drag on all the surface
drag_torque = T_aero_1 + T_aero_2 + T_aero_3 + T_aero_4 + T_aero_5 + T_aero_5 + T_aero_6;

% We want it in components
drag_torque_1 = drag_torque(1);
drag_torque_2 = drag_torque(2);
drag_torque_3 = drag_torque(3);

end

== matlab function Lab_5/Disturbance Torques/Areodynamic Drag Torque Calculator /MATLAB Function1 ==
  data: r input; rho output; R_e input
function rho = density_calculator(r,R_e)
%#codegen
% Exponential model for computing density

h = norm(r') - R_e;


H = 0;
h0 = 0;
rho_0 = 0; 
rho = 0;

if h > 200 && h <= 250
    H = 38.5;
    h0 = 200;
    rho_0 = 2.780e-10;
elseif h > 250 && h <= 300
    H = 46.9;
    h0 = 250;
    rho_0 = 7.248e-11;
elseif h > 300 && h <= 350
    H = 52.5;
    h0 = 300;
    rho_0 = 2.418e-11;
elseif h > 350 && h <= 400
    H = 56.4;
    h0 = 350;
    rho_0 = 9.158e-12;
elseif h > 400 && h <= 450
    H = 59.4;
    h0 = 400;
    rho_0 = 3.725e-12;
elseif h > 450 && h <= 500
    H = 62.2;
    h0 = 450;
    rho_0 = 1.585e-12;
elseif h > 500 && h <= 600
    H = 65.8;
    h0 = 500;
    rho_0 = 6.967e-13;
elseif h > 600 && h <= 700
    H = 79.0;
    h0 = 600;
    rho_0 = 1.454e-13;
elseif h > 700 && h <= 800
    H = 109.0;
    h0 = 700;
    rho_0 = 3.614e-14;
elseif h > 800 && h <= 900
    H = 164.0;
    h0 = 800;
    rho_0 = 1.170e-14;
elseif h >= 900 && h < 1000
    H = 225.0;
    h0 = 900;
    rho_0 = 5.245e-15;
elseif h >= 1000 
    H = 260.0;
    h0 = 1000;
    rho_0 = 3.019e-15;
end

rho = rho_0*exp(-(h-h0)/H);

== matlab function Lab_5/Disturbance Torques/Solar Radiation Pressure Torque Calculator/MATLAB Function ==
  data: r input; R_e input; S_b input; srp_torque_1 output; A_i input; dim input; rho_d input; srp_torque_2 output; srp_torque_3 output; rho_s input
function [srp_torque_1,srp_torque_2,srp_torque_3] = srp(r, R_e, S_b, A_i, dim, rho_d, rho_s)

% Define normal vectors
n_1 = [1 0 0];
n_2 = [0 1 0];
n_3 = [0 0 1];
n_4 = [-1 0 0];
n_5 = [0 -1 0];
n_6 = [0 0 -1];

% Dimensions 
w = dim(1);
l = dim(2);
h = dim(3);

% Sections 
A_i_1 = A_i(1);
A_i_2 = A_i(2);
A_i_3 = A_i(3);
A_i_4 = A_i(1);
A_i_5 = A_i(2);
A_i_6 = A_i(3);

% Distance between the center of pressure and the center of mass
% +0.1*rcg(da aggiungere)
r_1 = [h/2 0.1 0.1];
r_2 = [0.2 l/2 0.2];
r_3 = [0.4 0.4 w/2];
r_4 = [-h/2 0.1 0.1];
r_5 = [0.2 -l/2 0.2];
r_6 = [0.4 0.4 -w/2];

% Compute Solar Radiation Pressure
% Values taken from  Fundamentals of Spacecraft
% Attitude Determination and Control pag. 421
solar_flux = 1362;        % W/m^2
c = 299792458;            % m/s
P = solar_flux/c;         % Pa

S_b = S_b';

% Compute SRP on all the surface only if we are not shadowed by the Earth
if dot(r,S_b) < -sqrt((norm(r))^2 - R_e^2)
    srp_torque = [0 0 0];
else
    
    % Compute torque due to the solar radiation pressure only exposed faces.
    % If dot(S_b,n_i)) => 1 then the face is exposed othewise no.
    if dot(S_b,n_1) >= 0
        F_srp_1 = P*A_i_1*dot(S_b,n_1) * ((1-rho_s)*S_b + (2*rho_s*dot(S_b,n_1)+2/3*rho_d)*n_1);
        T_srp_1 = cross(r_1,F_srp_1);
    else
        T_srp_1 = [0 0 0];
    end
    
    if dot(S_b,n_2) >= 0
        F_srp_2 = P*A_i_2*dot(S_b,n_2) * ((1-rho_s)*S_b + (2*rho_s*dot(S_b,n_2)+2/3*rho_d)*n_2);
        T_srp_2 = cross(r_2,F_srp_2);
    else
        T_srp_2 = [0 0 0];
    end
    
    if dot(S_b,n_3) >= 0
        F_srp_3 = P*A_i_3*dot(S_b,n_3) * ((1-rho_s)*S_b + (2*rho_s*dot(S_b,n_3)+2/3*rho_d)*n_3);
        T_srp_3 = cross(r_3,F_srp_3);
    else
        T_srp_3 = [0 0 0];
    end
    
    if dot(S_b,n_4) >= 0
        F_srp_4 = P*A_i_4*dot(S_b,n_4) * ((1-rho_s)*S_b + (2*rho_s*dot(S_b,n_4)+2/3*rho_d)*n_4);
        T_srp_4 = cross(r_4,F_srp_4);
    else
        T_srp_4 = [0 0 0];
    end
    
    if dot(S_b,n_5) >= 0
        F_srp_5 = P*A_i_5*dot(S_b,n_5) * ((1-rho_s)*S_b + (2*rho_s*dot(S_b,n_5)+2/3*rho_d)*n_5);
        T_srp_5 = cross(r_5,F_srp_5);
    else
        T_srp_5 = [0 0 0];
    end
    
    if dot(S_b,n_6) >= 0
        F_srp_6 = P*A_i_6*dot(S_b,n_6) * ((1-rho_s)*S_b + (2*rho_s*dot(S_b,n_6)+2/3*rho_d)*n_6);
        T_aero_6 = cross(r_6,F_srp_6);
    else
        T_aero_6 = [0 0 0];
    end
    
    % Compute Solar Radiation Pressure on all surfaces
    srp_torque = T_srp_1 + T_srp_2 + T_srp_3 + T_srp_4 + T_srp_5 + T_srp_5 + T_aero_6;
end

% We want it in components
srp_torque_1 = srp_torque(1);
srp_torque_2 = srp_torque(2);
srp_torque_3 = srp_torque(3);

end

== matlab function Lab_5/Disturbance Torques/Magnetic Field Torque Calculator/Magnetic Field/MATLAB Function ==
  data: u input; y output
function y = norm2(u)

y = (norm(u))^2;

end

== matlab function Lab_5/Disturbance Torques/Magnetic Field Torque Calculator/Magnetic Field/MATLAB Function1 ==
  data: u input; y output
function y = norm5(u)

y = (norm(u))^5;

end

== matlab function Lab_5/Quaternion/Quaternion kinematics ==
  data: q input size=4; dq output size=4; omega input size=3
function dq = quat_kin(q, omega)
%#codegen
qnorm = sqrt(q(1)^2 + q(2)^2 + q(3)^2 + q(4)^2);
q = q./qnorm;
W = [ q(4) -q(3)  q(2) ;
      q(3)  q(4) -q(1) ;
     -q(2)  q(1)  q(4) ; 
     -q(1) -q(2) -q(3)];

dq = 0.5 * W * omega;

== matlab function Lab_5/Control/commanded quaternion matrix ==
  data: Q_C output; q_c input
function Q_C  = command_quaternion (q_c)
%#codegen

Q_C = [ q_c(4)  q_c(3)  -q_c(2) -q_c(1) ;
       -q_c(3)  q_c(4)   q_c(1) -q_c(2) ;
        q_c(2) -q_c(1)   q_c(4) -q_c(3) ; 
        q_c(1)  q_c(2)   q_c(3)  q_c(4) ];

end
